simulink model "SG__REF_I_104"  (R2022b)
settings: Solver=FixedStepAuto  StartTime=0.0  StopTime=Inf  RelTol=1e-3  EnableMultiTasking=on
model workspace (MAT data in the model file):
  N_trig = Simulink.Parameter
  N_trig.Value = 4
  N_trig.Description = 'number of samples for triggered pulse for recording'
  N_trig.DataType = 'auto'
  N_trig.Complexity = 'real'
  N_trig.Dimensions = [1 1]
  a_1 = Simulink.Parameter
  a_1.Value = [1 1 1]
  a_1.DataType = 'auto'
  a_1.Complexity = 'real'
  a_1.Dimensions = [1 3]
  b_1 = Simulink.Parameter
  b_1.Value = [0.5 0.5 0.5]
  b_1.DataType = 'auto'
  b_1.Complexity = 'real'
  b_1.Dimensions = [1 3]
  enable_source = Simulink.Parameter
  enable_source.Value = 0
  enable_source.DataType = 'boolean'
  enable_source.Complexity = 'real'
  enable_source.Dimensions = [1 1]
  freq_fin = Simulink.Parameter
  freq_fin.Value = 1200
  freq_fin.DataType = 'auto'
  freq_fin.Complexity = 'real'
  freq_fin.Dimensions = [1 1]
  freq_ini = Simulink.Parameter
  freq_ini.Value = 150
  freq_ini.DataType = 'auto'
  freq_ini.Complexity = 'real'
  freq_ini.Dimensions = [1 1]
  k_1 = Simulink.Parameter
  k_1.Value = [0 0 0]
  k_1.DataType = 'auto'
  k_1.Complexity = 'real'
  k_1.Dimensions = [1 3]
  rec = Simulink.Parameter
  rec.Value = 0
  rec.DataType = 'boolean'
  rec.Complexity = 'real'
  rec.Dimensions = [1 1]
  src_select = Simulink.Parameter
  src_select.Value = 0
  src_select.DataType = 'auto'
  src_select.Complexity = 'real'
  src_select.Dimensions = [1 1]
  sweep_gain = Simulink.Parameter
  sweep_gain.Value = 0.02
  sweep_gain.DataType = 'auto'
  sweep_gain.Complexity = 'real'
  sweep_gain.Dimensions = [1 1]
  tmax = Simulink.Parameter
  tmax.Value = 10
  tmax.DataType = 'auto'
  tmax.Complexity = 'real'
  tmax.Dimensions = [1 1]
  ts_rec = Simulink.Parameter
  ts_rec.Value = 0.0001
  ts_rec.DataType = 'auto'
  ts_rec.Complexity = 'real'
  ts_rec.Dimensions = [1 1]
undefined symbols (not defined in the file or in its folder): Ended, Single
libraries: speedgoatlib_IO104 x2, slrealtimeloglib x1, dspsigops x1
settings Model: SimulationMode=external  DataflowThreadingImplementation=Pthreads  Creator=padlewsk  LastModifiedBy=padlewsk
settings SolverCC: ConcurrentTasks=on  AlgebraicLoopSolver=TrustRegion  PositivePriorityOrder=on  AutoInsertRateTranBlk=on
settings DataIOCC: SaveFormat=StructureWithTime
settings OptimizationCC: GainParamInheritBuiltInType=on  RollThreshold=9  EfficientFloat2IntCast=on  SimCompilerOptimization=on
settings DebuggingCC: TasksWithSamePriorityMsg=none  UnconnectedInputMsg=warning  UnconnectedOutputMsg=warning  UnconnectedLineMsg=warning
settings HardwareCC: ProdBitPerLong=64  ProdLongLongMode=on  ProdHWDeviceType=Intel->x86-64 (Linux 64)
settings ModelReferenceCC: EnableRefExpFcnMdlSchedulingChecks=on  ModelReferenceNumInstancesAllowed=Single
settings RTWCC: Description=Simulink Real-Time  SystemTargetFile=slrealtime.tlc  TemplateMakefile=slrealtime_default_tmf  Toolchain=Simulink Real-Time Toolchain  BuildConfiguration=Faster Runs  CodeExecutionProfiling=on  TargetLang=C++

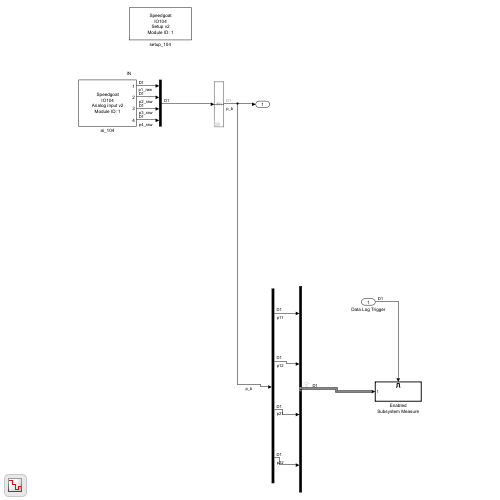
[thumbnail: Simulink's stored preview of the top-level diagram]
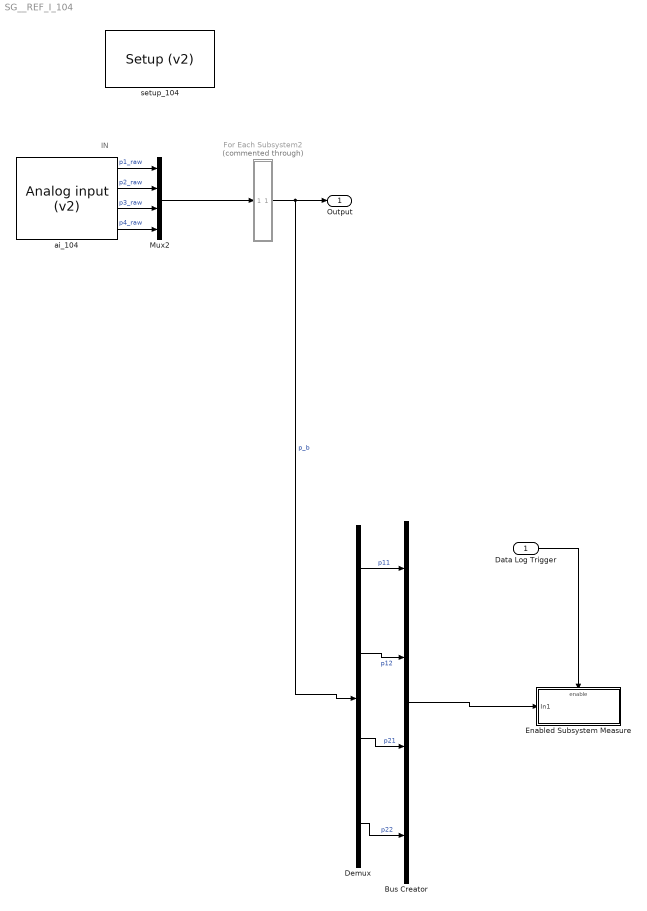
== system SG__REF_I_104 ==
  note: IN
  Data Log Trigger : Inport  OutDataTypeStr=boolean
  Bus Creator : BusCreator  Inputs=4
  Demux : Demux
  Enabled Subsystem Measure : Subsystem
  For Each Subsystem2 : Subsystem  Commented=through  TreatAsAtomicUnit=on
  Mux2 : Mux
  ai_104 : speedgoatlib_IO104/Analog input (v2)   parModuleId=1  parTs=ts  parPciSlot=-1  parAdChannels=[1,2,3,4]  parAdChannelsSorted=[1,2,3,4]  parAdRange1=+-2.5V  parAdRange2=+-2.5V  parAdCoupling=Single-Ended  parAdFrameSize=1  parAdUseTrigger=off  parAdClockInitiator=Initiator  parAdSampleTime=9.920634921e-07  parTriggerInitiator=Initiator  parTriggerRate=4.161015625e-01
      settings: SourceProductName=Simulink Real-Time: Speedgoat I/O Blockset
  setup_104 : speedgoatlib_IO104/Setup (v2)   parPciSlot=-1  parModuleId=1  parTriggerInitiator=Initiator  parTriggerRate=4.161015625e-01  parCalibrate=off  parAdChannels=[1:4]  parAdRange1=+-2.5V  parAdRange2=+-2.5V  parAdCoupling=Single-Ended  parAdUseTrigger=off  parAdFrameSize=1  parAdClockInitiator=Initiator  parAdSampleTime=9.920634921e-07  parDaSimultaneous=on  parDaChannels=[1:4]  parDaChannelsSorted=[1,2,3,4]  parDaInitValue=[0]  parDaReset=[1]  parDaRange=+-10V  parDaUseTrigger=off  parDaFrameSize=1  parDaClockInitiator=Initiator  parDaSampleTime=9.920634921e-07  parDioByte0Dir=Outputs  parDioByte1Dir=Inputs  parDoChannels=[]  parDoInitValues=[0]  parDoReset=[1]  parDiChannels=[]
      settings: SourceProductName=Simulink Real-Time: Speedgoat I/O Blockset
  Output : Outport
  wires:
  ai_104/3 -> Mux2/3  "p3_raw"
  ai_104/2 -> Mux2/2  "p2_raw"
  Mux2/1 -> For Each Subsystem2/1(In1)
  ai_104/1 -> Mux2/1  "p1_raw"
  ai_104/4 -> Mux2/4  "p4_raw"
  For Each Subsystem2/1(Out1) -> Output/1, Demux/1  "p_b"
  Demux/2 -> Bus Creator/2  "p12"
  Demux/1 -> Bus Creator/1  "p11"
  Bus Creator/1 -> Enabled Subsystem Measure/1(In1)
  Demux/3 -> Bus Creator/3  "p21"
  Demux/4 -> Bus Creator/4  "p22"
  Data Log Trigger/1 -> Enabled Subsystem Measure/Enable

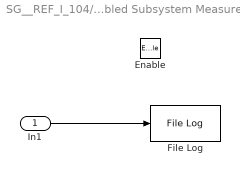
== system SG__REF_I_104/Enabled Subsystem Measure ==
  In1 : Inport
  Enable : EnablePort
  File Log : slrealtimeloglib/File Log  decimation=1  inputProcessing=Elements as channels (sample based)
  wires:
  In1/1 -> File Log/1

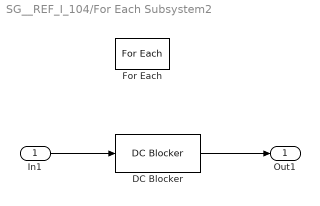
== system SG__REF_I_104/For Each Subsystem2 ==
  In1 : Inport  Partition=on  PartitionDimension=1  PartitionWidth=1  PartitionOffset=0
  DC Blocker : dspsigops/DC Blocker  Algorithm=FIR  NormalizedBandwidth=0.001  Length=50  Order=6  SimulateUsing=Code generation
      settings: LibrarySourceBlock=dsphdlsupportsigops/DC Blocker
  For Each : ForEach  DisableCoverage=on
  Out1 : Outport  ConcatenationDimension=1
  wires:
  In1/1 -> DC Blocker/1
  DC Blocker/1 -> Out1/1
